simulink model "simulink_sis_sus_auto"  (R2025a)
settings: Solver=VariableStepAuto  StartTime=0.0  StopTime=10.0  RelTol=1e-3
InitFcn:
  | m1=290
  | b1=1000
  | m2=59
  | k1=16182
  | f=0
  | k2=19000

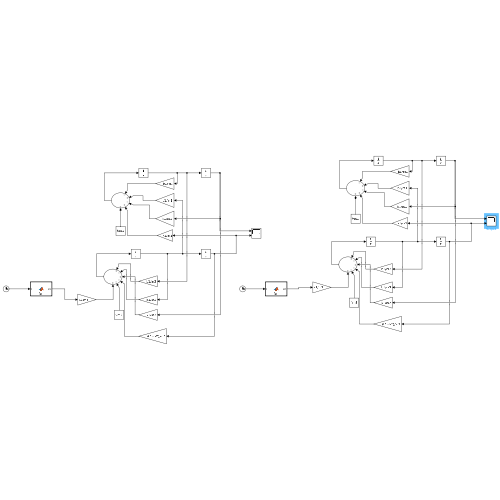
[thumbnail: Simulink's stored preview of the top-level diagram]
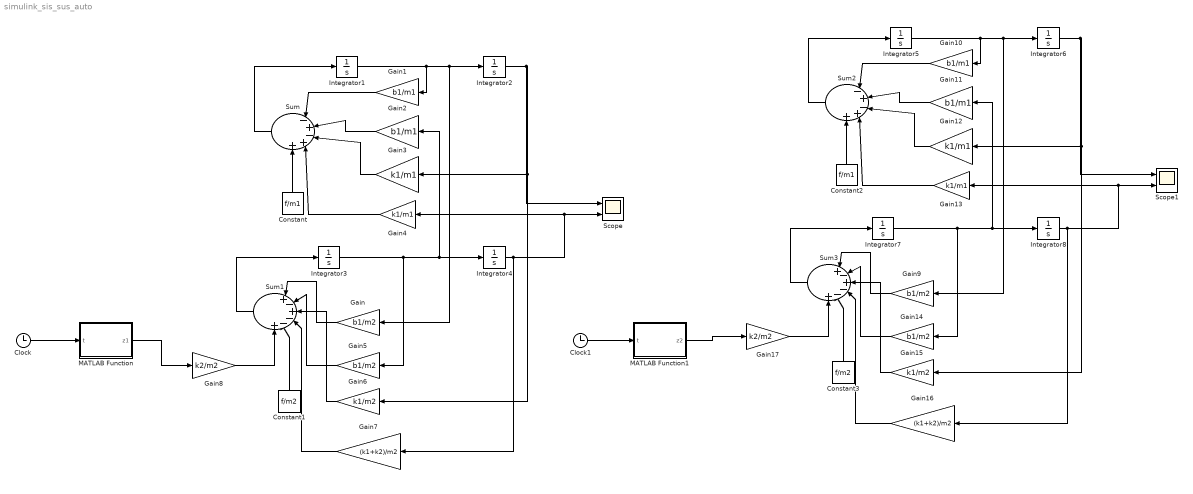
== system simulink_sis_sus_auto ==
  Clock : Clock
  Clock1 : Clock
  Constant : Constant  Value=f/m1
  Constant1 : Constant  Value=f/m2
  Constant2 : Constant  Value=f/m1
  Constant3 : Constant  Value=f/m2
  Gain{,5,9,14} (4 alike) : Gain  Gain=b1/m2
  Gain{1..2,10..11} (4 alike) : Gain  Gain=b1/m1
  Gain{3..4,12..13} (4 alike) : Gain  Gain=k1/m1
  Gain15 : Gain  Gain=k1/m2
  Gain16 : Gain  Gain=(k1+k2)/m2
  Gain17 : Gain  Gain=k2/m2
  Gain6 : Gain  Gain=k1/m2
  Gain7 : Gain  Gain=(k1+k2)/m2
  Gain8 : Gain  Gain=k2/m2
  Integrator{1..8} (8 alike) : Integrator
  MATLAB Function : MATLAB Function  TreatAsAtomicUnit=on
  MATLAB Function1 : MATLAB Function  TreatAsAtomicUnit=on
  Scope : Scope  NumInputPorts=2
      settings: ActiveDisplayYMinimum=-0.0702461517887558  ActiveDisplayYMaximum=0.080568748725473968
  Scope1 : Scope  NumInputPorts=2
      settings: ActiveDisplayYMinimum=-0.022694931008415738  ActiveDisplayYMaximum=0.013877191388818013
  Sum : Sum  Inputs=|-+-++
  Sum1 : Sum  Inputs=|+-+--+
  Sum2 : Sum  Inputs=|-+-++
  Sum3 : Sum  Inputs=|+-+--+
  wires:
  Integrator1/1 -> Gain1/1, Gain/1, Integrator2/1
  Sum/1 -> Integrator1/1
  Integrator2/1 -> Scope/1, Gain6/1, Gain3/1
  Gain1/1 -> Sum/1
  Gain2/1 -> Sum/2
  Sum1/1 -> Integrator3/1
  Integrator3/1 -> Gain5/1, Gain2/1, Integrator4/1
  Integrator4/1 -> Gain7/1, Gain4/1, Scope/2
  Gain3/1 -> Sum/3
  Gain4/1 -> Sum/4
  Constant/1 -> Sum/5
  Gain/1 -> Sum1/1
  Gain5/1 -> Sum1/2
  Gain6/1 -> Sum1/3
  Gain7/1 -> Sum1/4
  Constant1/1 -> Sum1/5
  Gain8/1 -> Sum1/6
  Clock/1 -> MATLAB Function/1(t)
  MATLAB Function/1(z1) -> Gain8/1
  Gain17/1 -> Sum3/6
  Integrator5/1 -> Gain10/1, Gain9/1, Integrator6/1
  Constant3/1 -> Sum3/5
  Gain16/1 -> Sum3/4
  Gain10/1 -> Sum2/1
  Sum2/1 -> Integrator5/1
  Sum3/1 -> Integrator7/1
  Integrator6/1 -> Scope1/1, Gain15/1, Gain12/1
  Integrator8/1 -> Gain16/1, Gain13/1, Scope1/2
  Constant2/1 -> Sum2/5
  Gain12/1 -> Sum2/3
  Gain11/1 -> Sum2/2
  Gain15/1 -> Sum3/3
  Integrator7/1 -> Gain14/1, Gain11/1, Integrator8/1
  Gain13/1 -> Sum2/4
  Gain9/1 -> Sum3/1
  Gain14/1 -> Sum3/2
  Clock1/1 -> MATLAB Function1/1(t)
  MATLAB Function1/1(z2) -> Gain17/1

== matlab function simulink_sis_sus_auto/MATLAB Function ==
  data: t input; z1 output
function z1 = fcn(t)
z1= 0.05*sin(0.5*pi*t)

== matlab function simulink_sis_sus_auto/MATLAB Function1 ==
  data: t input; z2 output
function z2 = fcn(t)
z2=0.05*sin(20*pi*t)
